simulink model "uvms_total"  (Simulink 8.1)
settings: Solver=ode23  StartTime=0.0  StopTime=2  FixedStep=dt  RelTol=1e-4
values from neighbouring files (symbols this model uses):
  DH = struct('a',zeros(n,1),'d',zeros(n,1),'alpha',zeros(n,1))    [init.m]
  dt = 0.01    [run_simulation.m]
undefined symbols (not defined in the file or in its folder): ee_pose_init, ee_pose_quaternion_init, KinematicControlParameters, Kinetics_Parameters, max_zeta, q_init, QLimits, reference_system_matrix_inv, reference_system_zeta_matrix_inv, V_current, vehicle_position_init, vehicle_quaternion_init, VV_States
(part 1 of 2)
settings Model: Creator=simena  LastModifiedBy=simena  SimulationMode=accelerator
settings SolverCC: ZeroCrossControl=DisableAll
settings DataIOCC: InspectSignalLogs=on
settings OptimizationCC: SimCompilerOptimization=On
settings DebuggingCC: AlgebraicLoopMsg=error  UnderspecifiedInitializationDetection=Simplified  FcnCallInpInsideContextMsg=EnableAllAsWarning
settings SFSimCC: SFSimEnableDebug=off
settings GRTTargetCC: CombineOutputUpdateFcns=on  GRTInterface=off

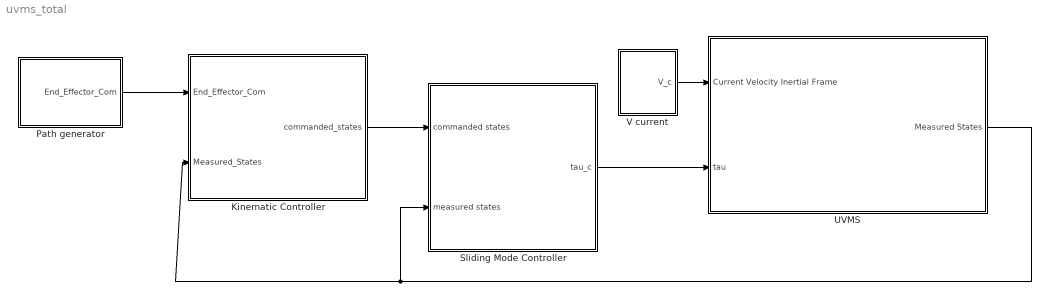
== system uvms_total ==
  Kinematic Controller : Subsystem
  Path generator : Subsystem
  Sliding Mode Controller : Subsystem
  UVMS : Subsystem
  V current : Subsystem
  wires:
  Sliding Mode Controller/1(tau_c) -> UVMS/2(tau)
  UVMS/1(Measured States) -> Sliding Mode Controller/2(measured states), Kinematic Controller/2(Measured_States)
  V current/1(V_c) -> UVMS/1(Current Velocity Inertial Frame)
  Path generator/1(End_Effector_Com) -> Kinematic Controller/1(End_Effector_Com)
  Kinematic Controller/1(commanded_states) -> Sliding Mode Controller/1(commanded states)

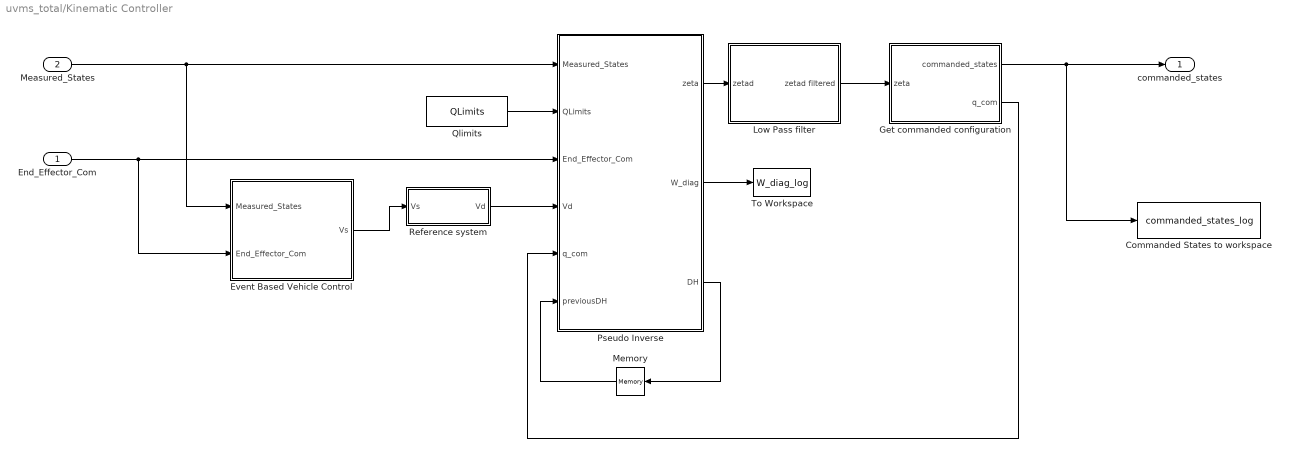
== system uvms_total/Kinematic Controller ==
  End_Effector_Com : Inport
  Measured_States : Inport  Port=2
  Commanded States to workspace : ToWorkspace  VariableName=commanded_states_log  SampleTime=dt  SaveFormat=Timeseries
  Event Based Vehicle Control : Subsystem
  Get commanded configuration : Subsystem  TreatAsAtomicUnit=on
  Low Pass filter : Subsystem
  Memory : Memory
  Pseudo Inverse : MATLAB Function  TreatAsAtomicUnit=on
  Qlimits : Constant  Value=QLimits  OutDataTypeStr=Bus: qlimits_bus
  Reference system : Subsystem
  To Workspace : ToWorkspace  VariableName=W_diag_log  SampleTime=dt  SaveFormat=Timeseries
  commanded_states : Outport
  wires:
  Qlimits/1 -> Pseudo Inverse/2(QLimits)
  Memory/1 -> Pseudo Inverse/6(previousDH)
  Event Based Vehicle Control/1(Vs) -> Reference system/1(Vs)
  Pseudo Inverse/2(W_diag) -> To Workspace/1
  Pseudo Inverse/3(DH) -> Memory/1
  Pseudo Inverse/1(zeta) -> Low Pass filter/1(zetad)
  Measured_States/1 -> Pseudo Inverse/1(Measured_States), Event Based Vehicle Control/1(Measured_States)
  Reference system/1(Vd) -> Pseudo Inverse/4(Vd)
  Get commanded configuration/2(q_com) -> Pseudo Inverse/5(q_com)
  Low Pass filter/1(zetad filtered) -> Get commanded configuration/1(zeta)
  Get commanded configuration/1(commanded_states) -> commanded_states/1, Commanded States to workspace/1
  End_Effector_Com/1 -> Pseudo Inverse/3(End_Effector_Com), Event Based Vehicle Control/2(End_Effector_Com)

== system uvms_total/Path generator ==
  EE velocity in frame 0 to EE velocity in frame e : MATLAB Function  TreatAsAtomicUnit=on
  End Effector2 : Subsystem
  From Workspace : FromWorkspace  VariableName=ee_traj_input  SampleTime=0
  To Workspace : ToWorkspace  VariableName=Ee_com_log  SampleTime=dt  SaveFormat=Timeseries
  End_Effector_Com : Outport
  wires:
  From Workspace/1 -> EE velocity in frame 0 to EE velocity in frame e/2(V0)  "v_ee_c_0"
  End Effector2/2(End Effector) -> End_Effector_Com/1, To Workspace/1
  EE velocity in frame 0 to EE velocity in frame e/1(Vb) -> End Effector2/1(v_ee_com)  "v_ee_c"
  End Effector2/1(ee_pose_euler) -> EE velocity in frame 0 to EE velocity in frame e/1(pose)

== system uvms_total/Sliding Mode Controller ==
  commanded states : Inport
  measured states : Inport  Port=2
  To Workspace1 : ToWorkspace  VariableName=tau_log  SampleTime=dt  SaveFormat=Timeseries
  sliding mode 2 : Subsystem
  tau_c : Outport
  wires:
  sliding mode 2/1(tau) -> To Workspace1/1, tau_c/1
  measured states/1 -> sliding mode 2/1(measured states)
  commanded states/1 -> sliding mode 2/2(commanded states)

== system uvms_total/UVMS ==
  Current Velocity Inertial Frame : Inport
  tau : Inport  Port=2
  Kinetics : Subsystem
      settings: MinAlgLoopOccurrences=on
  Log Measured States : Subsystem
  Measured States : Outport
  wires:
  tau/1 -> Kinetics/1(tau)
  Current Velocity Inertial Frame/1 -> Kinetics/2(Current Inertial Frame)
  Kinetics/1(measured_states) -> Log Measured States/1(measured_states), Measured States/1, Kinetics/3(Measured_States)

== system uvms_total/V current ==
  Current : Constant  Value=V_current
  V_c : Outport
  wires:
  Current/1 -> V_c/1

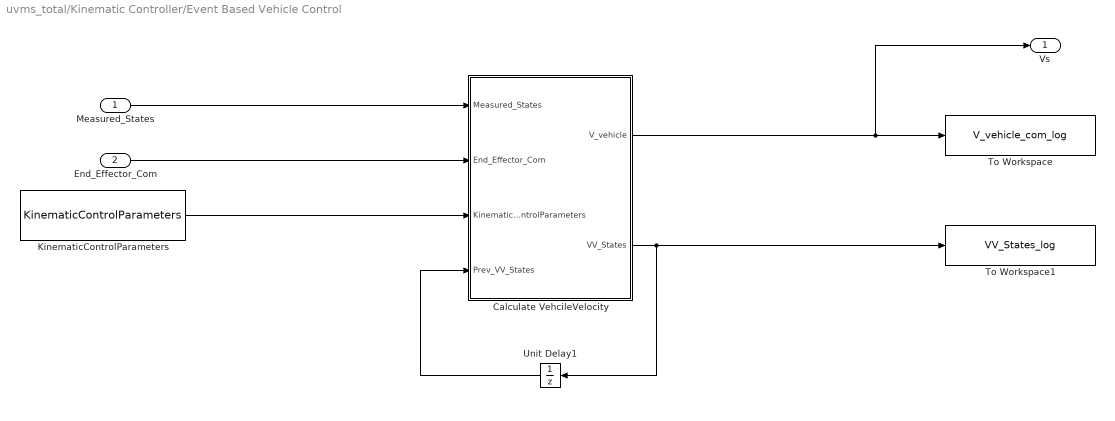
== system uvms_total/Kinematic Controller/Event Based Vehicle Control ==
  Measured_States : Inport
  End_Effector_Com : Inport  Port=2
  Calculate VehcileVelocity : MATLAB Function  TreatAsAtomicUnit=on  SystemSampleTime=dt
  KinematicControlParameters : Constant  Value=KinematicControlParameters  OutDataTypeStr=Bus: kinematicControlParameters_bus
  To Workspace : ToWorkspace  VariableName=V_vehicle_com_log  SampleTime=dt  SaveFormat=Timeseries
  To Workspace1 : ToWorkspace  VariableName=VV_States_log  SampleTime=dt  SaveFormat=Timeseries
  Unit Delay1 : UnitDelay  InitialCondition=VV_States  SampleTime=-1
  Vs : Outport
  wires:
  Unit Delay1/1 -> Calculate VehcileVelocity/4(Prev_VV_States)
  Measured_States/1 -> Calculate VehcileVelocity/1(Measured_States)
  End_Effector_Com/1 -> Calculate VehcileVelocity/2(End_Effector_Com)
  Calculate VehcileVelocity/2(VV_States) -> To Workspace1/1, Unit Delay1/1
  KinematicControlParameters/1 -> Calculate VehcileVelocity/3(KinematicControlParameters)
  Calculate VehcileVelocity/1(V_vehicle) -> Vs/1, To Workspace/1

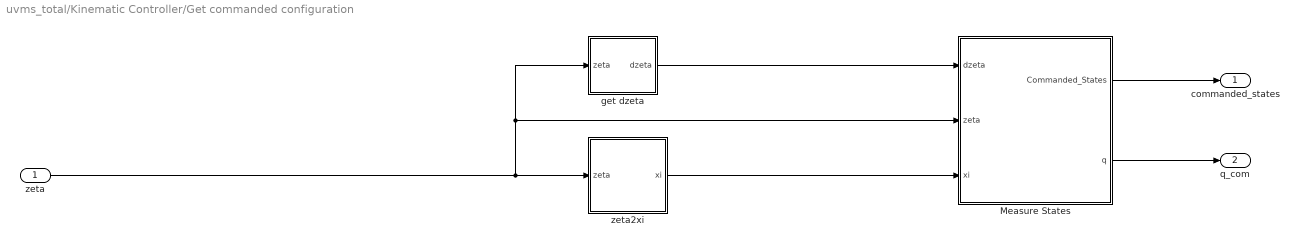
== system uvms_total/Kinematic Controller/Get commanded configuration ==
  zeta : Inport
  Measure States : MATLAB Function  TreatAsAtomicUnit=on
  get dzeta : Subsystem
  zeta2xi : Subsystem
  commanded_states : Outport
  q_com : Outport  Port=2
  wires:
  Measure States/1(Commanded_States) -> commanded_states/1
  zeta/1 -> zeta2xi/1(zeta), Measure States/2(zeta), get dzeta/1(zeta)
  get dzeta/1(dzeta) -> Measure States/1(dzeta)
  Measure States/2(q) -> q_com/1
  zeta2xi/1(xi) -> Measure States/3(xi)

== system uvms_total/Kinematic Controller/Low Pass filter ==
  zetad : Inport
  Integrator : Integrator
  Sum : Sum  Inputs=+-
  time constants : Gain  Gain=reference_system_zeta_matrix_inv  Multiplication=Matrix(K*u)
  zetad filtered : Outport
  wires:
  Sum/1 -> time constants/1
  Integrator/1 -> Sum/2, zetad filtered/1
  time constants/1 -> Integrator/1
  zetad/1 -> Sum/1

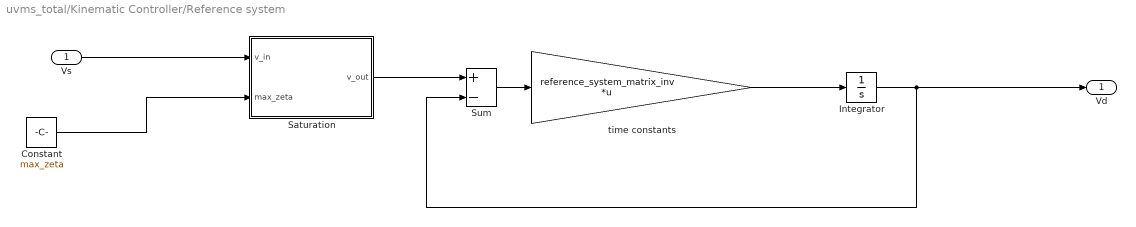
== system uvms_total/Kinematic Controller/Reference system ==
  Vs : Inport
  Constant : Constant  Value=max_zeta
  Integrator : Integrator  InitialCondition=zeros(6,1)
  Saturation : MATLAB Function  TreatAsAtomicUnit=on
  Sum : Sum  Inputs=+-
  time constants : Gain  Gain=reference_system_matrix_inv  Multiplication=Matrix(K*u)
  Vd : Outport
  wires:
  Sum/1 -> time constants/1
  Constant/1 -> Saturation/2(max_zeta)
  time constants/1 -> Integrator/1
  Saturation/1(v_out) -> Sum/1
  Vs/1 -> Saturation/1(v_in)
  Integrator/1 -> Vd/1, Sum/2

== system uvms_total/Path generator/End Effector2 ==
  v_ee_com : Inport
  MATLAB Function1 : MATLAB Function  TreatAsAtomicUnit=on
  twist2pose_euler : Subsystem
  twist2pose_quaternions : Subsystem
  ee_pose_euler : Outport
  End Effector : Outport  Port=2
  wires:
  MATLAB Function1/1(End_Effector_Com) -> End Effector/1
  v_ee_com/1 -> MATLAB Function1/1(velocity), twist2pose_euler/1(v_ee), twist2pose_quaternions/1(v_ee)
  twist2pose_euler/1(ee_pose) -> ee_pose_euler/1
  twist2pose_quaternions/1(ee_pose) -> MATLAB Function1/2(pose)

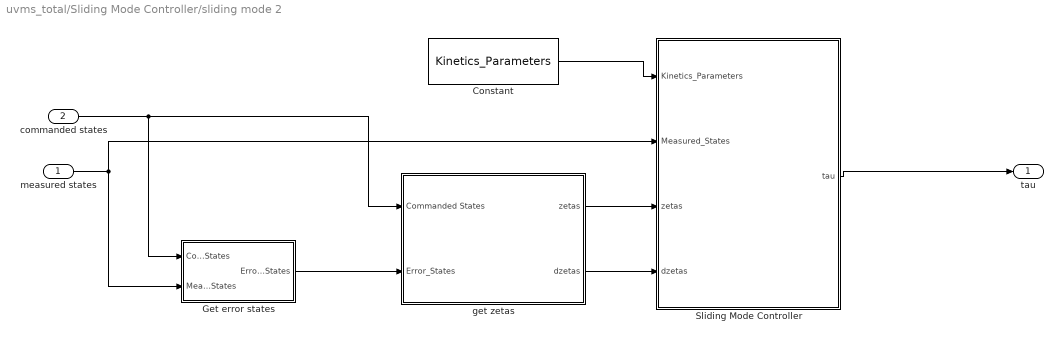
== system uvms_total/Sliding Mode Controller/sliding mode 2 ==
  measured states : Inport
  commanded states : Inport  Port=2
  Constant : Constant  Value=Kinetics_Parameters  OutDataTypeStr=Bus: kinetics_bus
  Get error states : Subsystem
  Sliding Mode Controller : MATLAB Function  TreatAsAtomicUnit=on
  get zetas : Subsystem
  tau : Outport
  wires:
  Constant/1 -> Sliding Mode Controller/1(Kinetics_Parameters)
  Sliding Mode Controller/1(tau) -> tau/1
  get zetas/1(zetas) -> Sliding Mode Controller/3(zetas)
  get zetas/2(dzetas) -> Sliding Mode Controller/4(dzetas)
  commanded states/1 -> get zetas/1(Commanded States), Get error states/1(Commanded States)
  measured states/1 -> Sliding Mode Controller/2(Measured_States), Get error states/2(Measured States)
  Get error states/1(Error States) -> get zetas/2(Error_States)

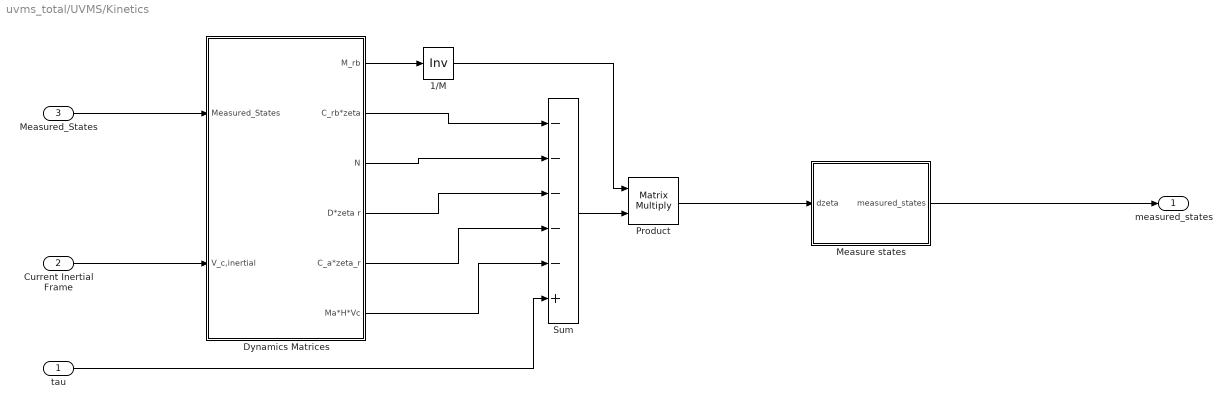
== system uvms_total/UVMS/Kinetics ==
  tau : Inport
  Current Inertial Frame : Inport  Port=2
  Measured_States : Inport  Port=3
  1/M : Product  Inputs=/  Multiplication=Matrix(*)
  Dynamics Matrices : Subsystem
  Measure states : Subsystem  TreatAsAtomicUnit=on
      settings: MinAlgLoopOccurrences=on
  Product : Product  Multiplication=Matrix(*)  RndMeth=Zero
  Sum : Sum  Inputs=-----+
  measured_states : Outport
  wires:
  Dynamics Matrices/1(M_rb) -> 1/M/1
  Sum/1 -> Product/2
  Product/1 -> Measure states/1(dzeta)
  Measure states/1(measured_states) -> measured_states/1
  1/M/1 -> Product/1
  Current Inertial Frame/1 -> Dynamics Matrices/2(V_c,inertial)
  Dynamics Matrices/2(C_rb*zeta) -> Sum/1
  Dynamics Matrices/3(N) -> Sum/2
  Dynamics Matrices/4(D*zeta r) -> Sum/3
  Dynamics Matrices/5(C_a*zeta_r) -> Sum/4
  Dynamics Matrices/6(Ma*H*Vc) -> Sum/5
  tau/1 -> Sum/6
  Measured_States/1 -> Dynamics Matrices/1(Measured_States)

== system uvms_total/UVMS/Log Measured States ==
  measured_states : Inport
  To Workspace1 : ToWorkspace  VariableName=measured_states_log  SampleTime=dt  SaveFormat=Timeseries
  wires:
  measured_states/1 -> To Workspace1/1

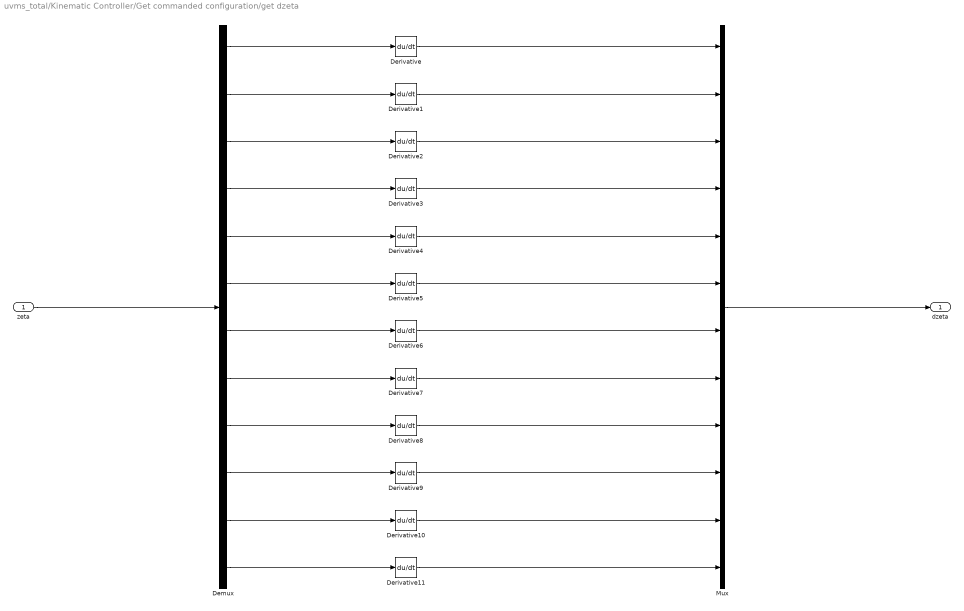
== system uvms_total/Kinematic Controller/Get commanded configuration/get dzeta ==
  zeta : Inport
  Demux : Demux  Outputs=12
  Derivative{,1..11} (12 alike) : Derivative
  Mux : Mux  Inputs=12
  dzeta : Outport
  wires:
  Demux/1 -> Derivative/1
  zeta/1 -> Demux/1
  Derivative/1 -> Mux/1
  Demux/2 -> Derivative1/1
  Demux/3 -> Derivative2/1
  Demux/4 -> Derivative3/1
  Demux/5 -> Derivative4/1
  Demux/6 -> Derivative5/1
  Demux/7 -> Derivative6/1
  Demux/8 -> Derivative7/1
  Demux/9 -> Derivative8/1
  Demux/10 -> Derivative9/1
  Demux/11 -> Derivative10/1
  Demux/12 -> Derivative11/1
  Derivative1/1 -> Mux/2
  Derivative2/1 -> Mux/3
  Derivative3/1 -> Mux/4
  Derivative4/1 -> Mux/5
  Derivative5/1 -> Mux/6
  Derivative6/1 -> Mux/7
  Derivative7/1 -> Mux/8
  Derivative8/1 -> Mux/9
  Derivative9/1 -> Mux/10
  Derivative10/1 -> Mux/11
  Derivative11/1 -> Mux/12
  Mux/1 -> dzeta/1

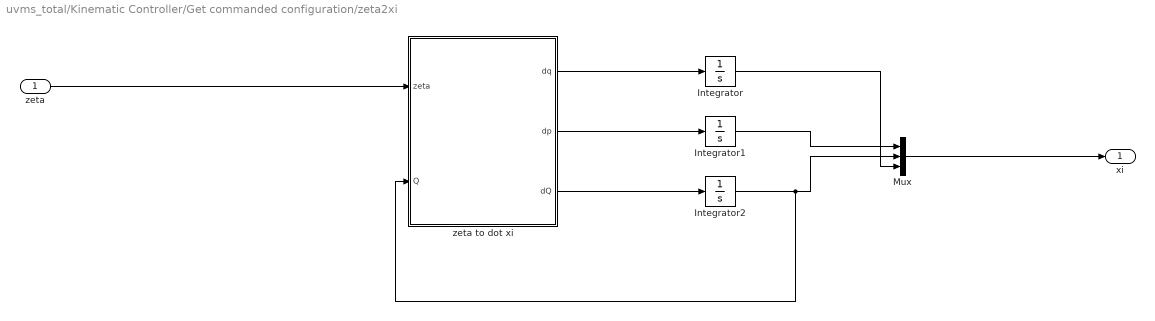
== system uvms_total/Kinematic Controller/Get commanded configuration/zeta2xi ==
  zeta : Inport
  Integrator : Integrator  InitialCondition=q_init
  Integrator1 : Integrator  InitialCondition=vehicle_position_init
  Integrator2 : Integrator  InitialCondition=vehicle_quaternion_init
  Mux : Mux  Inputs=3
  zeta to dot xi : MATLAB Function  TreatAsAtomicUnit=on
  xi : Outport
  wires:
  zeta to dot xi/1(dq) -> Integrator/1
  zeta to dot xi/2(dp) -> Integrator1/1
  zeta to dot xi/3(dQ) -> Integrator2/1
  zeta/1 -> zeta to dot xi/1(zeta)
  Mux/1 -> xi/1
  Integrator1/1 -> Mux/1
  Integrator2/1 -> Mux/2, zeta to dot xi/2(Q)
  Integrator/1 -> Mux/3

== system uvms_total/Path generator/End Effector2/twist2pose_euler ==
  v_ee : Inport
  Demux : Demux  Outputs=2
  Integrator : Integrator  InitialCondition=ee_pose_init
  Mux : Mux  Inputs=2
  body2eulervel : MATLAB Function  TreatAsAtomicUnit=on  SystemSampleTime=dt
  ee_pose : Outport
  wires:
  v_ee/1 -> body2eulervel/1(ee_velocity_twist)
  body2eulervel/1(ee_rates) -> Integrator/1
  Integrator/1 -> Demux/1
  Demux/2 -> body2eulervel/2(euler_angles_ee), Mux/2  "ee_angle"
  Demux/1 -> Mux/1  "ee_pos"
  Mux/1 -> ee_pose/1

== system uvms_total/Path generator/End Effector2/twist2pose_quaternions ==
  v_ee : Inport
  Integrator : Integrator  InitialCondition=ee_pose_quaternion_init
  MATLAB Function : MATLAB Function  TreatAsAtomicUnit=on
  body2quat : MATLAB Function  TreatAsAtomicUnit=on  SystemSampleTime=dt
  ee_pose : Outport
  wires:
  v_ee/1 -> body2quat/1(ee_velocity_twist)
  body2quat/1(ee_rates) -> Integrator/1
  Integrator/1 -> MATLAB Function/1(poseIn)
  MATLAB Function/1(pose) -> ee_pose/1
  MATLAB Function/2(quaternion) -> body2quat/2(quat)

== system uvms_total/Sliding Mode Controller/sliding mode 2/Get error states ==
  Commanded States : Inport
  Measured States : Inport  Port=2
  Log Error States : Subsystem
  MATLAB Function : MATLAB Function  TreatAsAtomicUnit=on
  Error States : Outport
  wires:
  Commanded States/1 -> MATLAB Function/1(Commanded_States)
  Measured States/1 -> MATLAB Function/2(Measured_States)
  MATLAB Function/1(Error_States) -> Log Error States/1(measured_states), Error States/1

== system uvms_total/Sliding Mode Controller/sliding mode 2/get zetas ==
  Commanded States : Inport
  Error_States : Inport  Port=2
  Derivative : Derivative  CoefficientInTFapproximation=0.01
  get dot y : MATLAB Function  TreatAsAtomicUnit=on
  zetas : Outport
  dzetas : Outport  Port=2
  wires:
  Commanded States/1 -> get dot y/1(Commanded_States)
  Error_States/1 -> get dot y/2(Error_States)
  get dot y/1(zetas) -> zetas/1, Derivative/1
  Derivative/1 -> dzetas/1

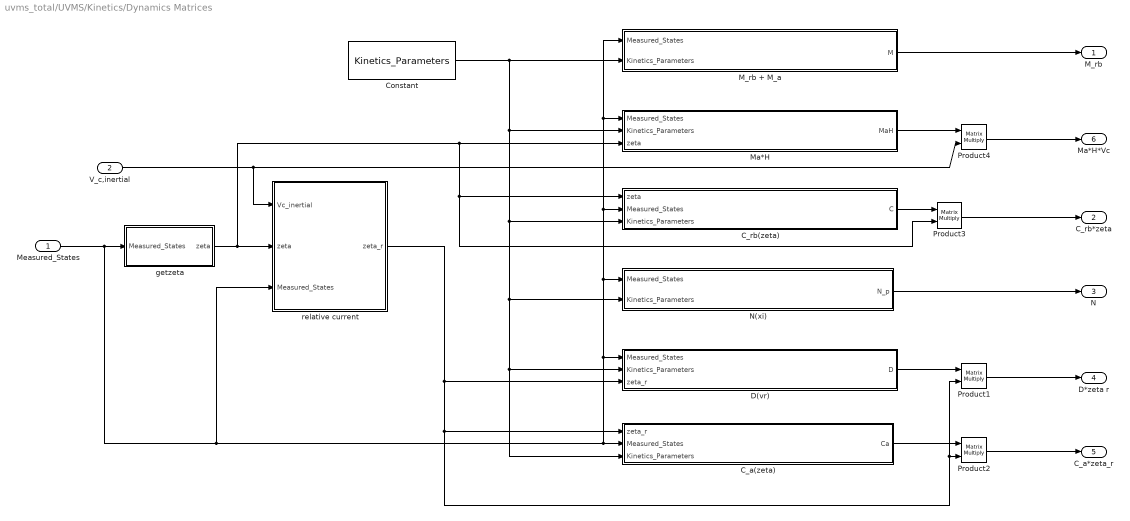
== system uvms_total/UVMS/Kinetics/Dynamics Matrices ==
  Measured_States : Inport
  V_c,inertial : Inport  Port=2
  C_a(zeta) : MATLAB Function  TreatAsAtomicUnit=on
  C_rb(zeta) : MATLAB Function  TreatAsAtomicUnit=on
  Constant : Constant  Value=Kinetics_Parameters  OutDataTypeStr=Bus: kinetics_bus
  D(vr) : MATLAB Function  TreatAsAtomicUnit=on
  M_rb + M_a : MATLAB Function  TreatAsAtomicUnit=on
  Ma*H : MATLAB Function  TreatAsAtomicUnit=on
  N(xi) : MATLAB Function  TreatAsAtomicUnit=on
  Product{1..4} (4 alike) : Product  Multiplication=Matrix(*)  RndMeth=Zero
  getzeta : MATLAB Function  TreatAsAtomicUnit=on
  relative current : MATLAB Function  TreatAsAtomicUnit=on
  M_rb : Outport
  C_rb*zeta : Outport  Port=2
  N : Outport  Port=3
  D*zeta r : Outport  Port=4
  C_a*zeta_r : Outport  Port=5
  Ma*H*Vc : Outport  Port=6
  wires:
  Product1/1 -> D*zeta r/1
  Product2/1 -> C_a*zeta_r/1
  Product3/1 -> C_rb*zeta/1
  M_rb + M_a/1(M) -> M_rb/1
  Ma*H/1(MaH) -> Product4/1
  relative current/1(zeta_r) -> D(vr)/3(zeta_r), C_a(zeta)/1(zeta_r), Product2/2, Product1/2
  Measured_States/1 -> relative current/3(Measured_States), C_a(zeta)/2(Measured_States), D(vr)/1(Measured_States), N(xi)/1(Measured_States), C_rb(zeta)/2(Measured_States), Ma*H/1(Measured_States), M_rb + M_a/1(Measured_States), getzeta/1(Measured_States)
  Constant/1 -> M_rb + M_a/2(Kinetics_Parameters), Ma*H/2(Kinetics_Parameters), C_rb(zeta)/3(Kinetics_Parameters), N(xi)/2(Kinetics_Parameters), C_a(zeta)/3(Kinetics_Parameters), D(vr)/2(Kinetics_Parameters)
  C_rb(zeta)/1(C) -> Product3/1
  N(xi)/1(N_p) -> N/1
  D(vr)/1(D) -> Product1/1
  C_a(zeta)/1(Ca) -> Product2/1
  V_c,inertial/1 -> Product4/2, relative current/1(Vc_inertial)
  Product4/1 -> Ma*H*Vc/1
  getzeta/1(zeta) -> relative current/2(zeta), Ma*H/3(zeta), C_rb(zeta)/1(zeta), Product3/2

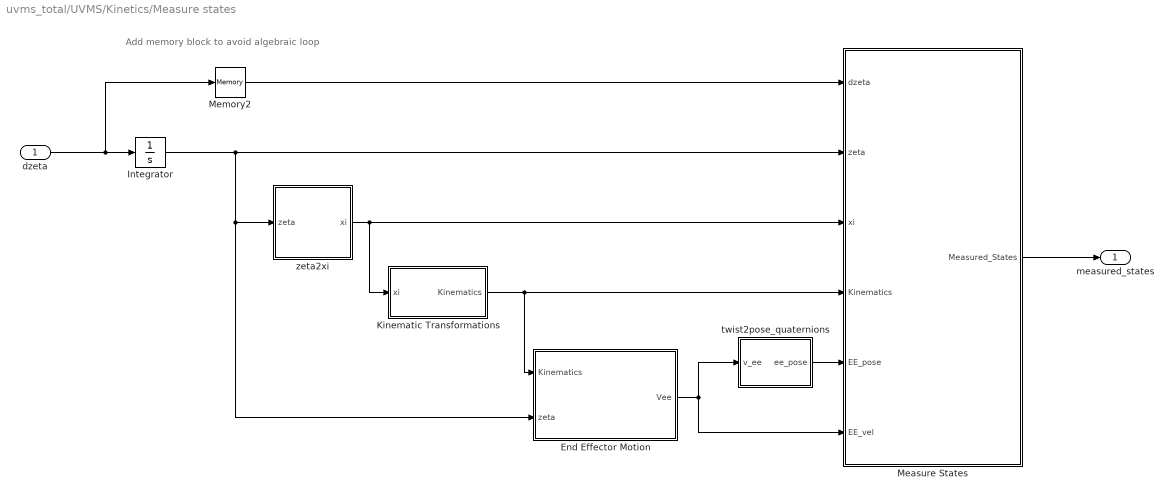
== system uvms_total/UVMS/Kinetics/Measure states ==
  note: Add memory block
      | to avoid algebraic
      | loop
  dzeta : Inport
  End Effector Motion : MATLAB Function  TreatAsAtomicUnit=on
  Integrator : Integrator
  Kinematic Transformations : Subsystem  SystemSampleTime=dt
      settings: MinAlgLoopOccurrences=on
  Measure States : MATLAB Function  TreatAsAtomicUnit=on
  Memory2 : Memory
  twist2pose_quaternions : Subsystem
  zeta2xi : Subsystem
  measured_states : Outport
  wires:
  Measure States/1(Measured_States) -> measured_states/1
  zeta2xi/1(xi) -> Measure States/3(xi), Kinematic Transformations/1(xi)
  Memory2/1 -> Measure States/1(dzeta)
  dzeta/1 -> Integrator/1, Memory2/1
  Integrator/1 -> End Effector Motion/2(zeta), zeta2xi/1(zeta), Measure States/2(zeta)
  twist2pose_quaternions/1(ee_pose) -> Measure States/5(EE_pose)
  End Effector Motion/1(Vee) -> Measure States/6(EE_vel), twist2pose_quaternions/1(v_ee)
  Kinematic Transformations/1(Kinematics) -> End Effector Motion/1(Kinematics), Measure States/4(Kinematics)

== system uvms_total/Sliding Mode Controller/sliding mode 2/Get error states/Log Error States ==
  measured_states : Inport
  To Workspace1 : ToWorkspace  VariableName=Error_States_log  SampleTime=dt  SaveFormat=Timeseries
  wires:
  measured_states/1 -> To Workspace1/1

== system uvms_total/UVMS/Kinetics/Measure states/Kinematic Transformations ==
  xi : Inport
  DH parameters : Constant  Value=DH  OutDataTypeStr=Bus: DH_bus
  Jacobians : MATLAB Function  TreatAsAtomicUnit=on
  Transformations : MATLAB Function  TreatAsAtomicUnit=on
  Kinematics : Outport
  wires:
  DH parameters/1 -> Transformations/2(DH)  "DH"
  Transformations/1(Ti) -> Jacobians/1(Ti)
  Jacobians/1(Kinematics) -> Kinematics/1
  xi/1 -> Transformations/1(xi)

== system uvms_total/UVMS/Kinetics/Measure states/twist2pose_quaternions ==
  v_ee : Inport
  Integrator : Integrator  InitialCondition=ee_pose_quaternion_init
  MATLAB Function : MATLAB Function  TreatAsAtomicUnit=on
  body2quat : MATLAB Function  TreatAsAtomicUnit=on
  ee_pose : Outport
  wires:
  v_ee/1 -> body2quat/1(ee_velocity_twist)
  body2quat/1(ee_rates) -> Integrator/1
  Integrator/1 -> MATLAB Function/1(poseIn)
  MATLAB Function/1(pose) -> ee_pose/1
  MATLAB Function/2(quaternion) -> body2quat/2(quat)

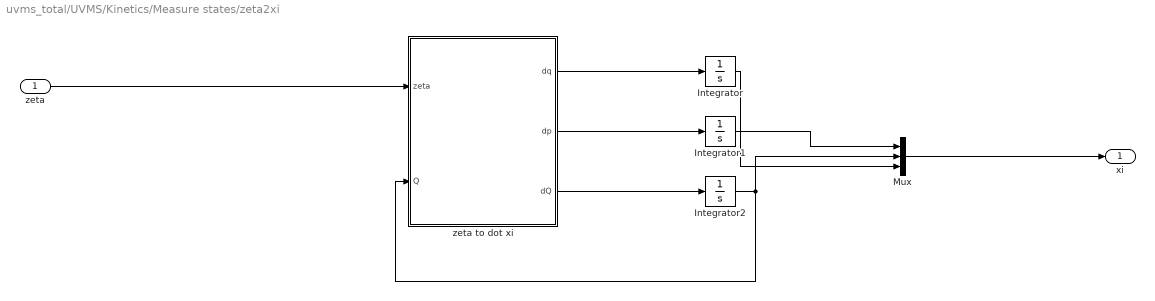
== system uvms_total/UVMS/Kinetics/Measure states/zeta2xi ==
  zeta : Inport
  Integrator : Integrator  InitialCondition=q_init
  Integrator1 : Integrator  InitialCondition=vehicle_position_init
  Integrator2 : Integrator  InitialCondition=vehicle_quaternion_init
  Mux : Mux  Inputs=3
  zeta to dot xi : MATLAB Function  TreatAsAtomicUnit=on  SystemSampleTime=dt
  xi : Outport
  wires:
  zeta to dot xi/1(dq) -> Integrator/1
  zeta to dot xi/2(dp) -> Integrator1/1
  zeta to dot xi/3(dQ) -> Integrator2/1
  zeta/1 -> zeta to dot xi/1(zeta)
  Integrator2/1 -> zeta to dot xi/2(Q), Mux/2
  Mux/1 -> xi/1
  Integrator1/1 -> Mux/1
  Integrator/1 -> Mux/3

== matlab function UVMS/Kinetics/Measure states/Kinematic Transformations/Jacobians ==
  data: Ti input Bus: Ti_bus; Kinematics output Bus: kin_bus
function Kinematics  = getJacobians(Ti)
%#codegen
    n=6;
    Ji = struct('Ji',zeros(n,n+6,n),'Je',zeros(n,n+6),'Jbe',zeros(n,n));
    Kinematics = struct('Ti', Ti, 'Ji',Ji);
    ji=zeros(6,6);
    for i=1:n
        ji=getji(Ti,i);
    
        Ji.Ji(:,:,i) = [Ti.Adgbi_inv(:,:,i), Ti.Adgbi_inv(:,:,i)*ji];
    end
    j6 = getje(Ti);
    Ji.Je = [Ti.Adgbe_inv, Ti.Adgbe_inv*j6];
    Ji.Jbe = Ti.Adgbe_inv*j6;
    Kinematics.Ji = Ji;
    Kinematics.Ti = Ti;
end




% return matrix Ji (see report)
function mat = getji(Ti,i)
    n=6;
    mat=zeros(6,6);
    Xii=[0,0,0,0,0,1]';
    mat(:,1)=eye(6)*Xii;
    for j=2:n
        if j<=i
            mat(:,j) = Ti.Adgbi(:,:,j-1)*Xii;
        end
    end

end

% return matrix Je (see report)
function mat = getje(Ti)
    n=6;
    mat=zeros(6,6);
    Xii=[0,0,0,0,0,1]';
    mat(:,1)=eye(6)*Xii;
    for i=2:(n-1)
        mat(:,i) = Ti.Adgbi(:,:,i-1)*Xii;
    end
    mat(:,6) = Ti.Adgbe*Xii;

end

== matlab function UVMS/Kinetics/Measure states/Kinematic Transformations/Transformations ==
  data: xi input double; DH input Bus: DH_bus; Ti output Bus: Ti_bus
function Ti = getTransformations(xi,DH)
%#codegen
% Return transformations, rotations, positions and adjoint matrices for
% robot links
% Tbi.gbi(:,:,i) is the transformation from b to i etc
    n = 6;    % number of links
    %xi = Measured_States.xi;
    q = xi(8:13);
    eta = xi(1:7);
    Q = eta(4:7);
    x = eta(1:3);
    Ti = struct('g0b',zeros(4,4),'g0i',zeros(4,4,n),'R0i', zeros(3,3,n),'R0b',zeros(3,3),'p0i', zeros(3,1,n),  'Adg0i',zeros(6,6,n),'Adg0i_inv',zeros(6,6,n),   ...
    'gbi',zeros(4,4,n),'Rbi', zeros(3,3,n),'pbi', zeros(3,1,n),'Adgbi',zeros(6,6,n),'Adgbi_inv',zeros(6,6,n),...
    'g6e', eye(4) ,'g0e',zeros(4,4),'R0e', zeros(3,3),'p0e', zeros(3,1),  'Adg0e',zeros(6,6),'Adg0e_inv',zeros(6,6),   ...
    'gbe',zeros(4,4),'Rbe', zeros(3,3),'pbe', zeros(3,1),'Adgbe',zeros(6,6),'Adgbe_inv',zeros(6,6) ...
    );
        
    Ti.g0b = eta2g0b(eta);
    Ti.R0b = Ti.g0b(1:3,1:3);

    % initial matrices 
    g = eye(4);
    g0 = Ti.g0b;
    
    for xi = 1:n
       % transformations from frame b to frame i
       Ti.gbi(:,:,xi) = g*getHom(q,DH,xi);
       Ti.Rbi(:,:,xi) = getRot(Ti.gbi(:,:,xi));
       Ti.pbi(:,:,xi) = getPos(Ti.gbi(:,:,xi));
       Ti.Adgbi(:,:,xi) = getAdgbi(Ti.Rbi(:,:,xi), Ti.pbi(:,:,xi) );
       Ti.Adgbi_inv(:,:,xi) = getAdgbi_inv(Ti.Rbi(:,:,xi), Ti.pbi(:,:,xi) );
       g = Ti.gbi(:,:,xi);
       % transformations from frame 0 to frame i
       Ti.g0i(:,:,xi) = g0*getHom(q,DH,xi);
       Ti.R0i(:,:,xi) = getRot(Ti.g0i(:,:,xi));
       Ti.p0i(:,:,xi) = getPos(Ti.g0i(:,:,xi));
       Ti.Adg0i(:,:,xi) = getAdgbi(Ti.R0i(:,:,xi), Ti.p0i(:,:,xi) );
       Ti.Adg0i_inv(:,:,xi) = getAdgbi_inv(Ti.R0i(:,:,xi), Ti.p0i(:,:,xi) );
       g0 = Ti.g0i(:,:,xi);
    end
    
    % transformation from frame 0 to ee
    g0e = Ti.g0i(:,:,6)*Ti.g6e;
    Ti.g0e = g0e;
    Ti.R0e = getRot(g0e);
    Ti.p0e = getPos(g0e);
    Ti.Adg0e = getAdgbi(Ti.R0e, Ti.p0e );
    Ti.Adg0e_inv = getAdgbi_inv(Ti.R0e, Ti.p0e);
        
    % transformation from frame b to ee
    gbe = Ti.gbi(:,:,6)*Ti.g6e;
    Ti.gbe = gbe;
    Ti.Rbe = getRot(gbe);
    Ti.pbe = getPos(gbe);
    Ti.Adgbe = getAdgbi(Ti.Rbe , Ti.pbe );
    Ti.Adgbe_inv = getAdgbi_inv(Ti.Rbe , Ti.pbe );
        
 end

% homogenous transformation matrix - DH convention
% mat = Rot_z(theta)Trans_z(d)Trans_x(a)Rot_x(alpha)
function mat = getHom(q,DH,i)
    alpha = DH.alpha(i);
    a = DH.a(i);
    d = DH.d(i);
    theta = q(i);
    mat = eye(4);
    mat = [cos(theta), -sin(theta)*cos(alpha), sin(theta)*sin(alpha), a*cos(theta);
         sin(theta), cos(theta)*cos(alpha), -cos(theta)*sin(alpha), a*sin(theta);
         0, sin(alpha), cos(alpha), d;
         0,0,0,1
    ];
end

% extract position from homogenous 
% matrix
function vec = getPos(g)
    vec = g(1:3,4);
end

% extract rotation matrix-part out of
% homogenous matrix
function mat = getRot(g)
    mat = g(1:3,1:3);
end

function mat = getAdgbi(R,p)
    ps = skew(p);
    mat = [R , ps*R ; zeros(3,3), R ];
end

function mat = getAdgbi_inv(R,p)
    Rt = transpose(R);
    ps = skew(p);
    mat = [Rt , -Rt*ps ; zeros(3,3), Rt ];
end

function mat = eta2g0b(eta)
    R = Rquat(eta(4:7));
    pos = [eta(1); eta(2); eta(3)];
    mat = [R,pos;0,0,0,1];
end

%-----------------------------------------------
% get rotation matrix from quaternion
function R = Rquat(Q)
    tol = 5*1e-2;
    if abs(norm(Q)-1)>tol 
        Q
        norm(Q)
        error('norm(q) must be equal to 1 (in get transformations) Try decreasing sampling time');
    end
    eta = Q(1);
    eps = Q(2:4);
    S = skew(eps);
    R = eye(3) + 2*eta*S + 2*S^2;
end

== matlab function Kinematic Controller/Pseudo Inverse ==
  data: Measured_States input Bus: measured_states_bus; QLimits input Bus: qlimits_bus; zeta output double size=12; W_diag output double; End_Effector_Com input double; Vd input double; q_com input double; previousDH input double; DH output double size=12,12
function [zeta, W_diag, DH] = getZeta(Measured_States, QLimits, End_Effector_Com, Vd , q_com , previousDH)
%
%  Vp is the primary task trajectory - end effector
%  Vs is the secondary task trajectory - vehicle
%
%#codegen
    Jp = Measured_States.Ji.Je;
    Js = [eye(6), zeros(6,6)];
    q = q_com;
    Vp = End_Effector_Com.velocity;
    [W, DH] = getW(q,previousDH,QLimits);
    JpInv = zeros(12,6);
    JsInv = zeros(12,6);
    JsInv(:,:) = Js' ; 
    JpInv(:,:) = W \ transpose(Jp) /((Jp /W) *transpose(Jp));
    I = eye(12);
    zeta = JpInv*(Vp  ) + ( I - JpInv*Jp) * JsInv * Vd;
    W_diag = diag(W);
end

% --------------------------------------------------------------------------
%   Returns the weighting matrix for use in the weighted pseudo inverse
% --------------------------------------------------------------------------
function [W, DH] = getW(q, previousDH,QLimits)
%#codegen    
% link joints
    DH =diag([zeros(1,6),zeros(1,6)]); % derivative of H matrix
    qmin = QLimits.qmin;
    qmax = QLimits.qmax;
    for i=1:6
        temp = (((qmax(i)-qmin(i)).^2)*(2*q(i)-qmax(i)-qmin(i))) ./ ((4*(qmax(i)-q(i)).^2) * ((q(i)-qmin(i)).^2));
        if (abs(temp) - abs(previousDH(i+6,i+6))) < 0 
            DH(i+6,i+6) = 0.97 * previousDH(i+6, i+6);
         else
            DH(i+6,i+6) = temp;
        end
   end
   % vehicle weights
   Kv = 4000;
   for i=1:6
      DH(i,i) =  Kv ;
   end
   W = eye(12);
   W = W + abs(DH);
   
end

== matlab function UVMS/Kinetics/Dynamics Matrices/M_rb + M_a ==
  data: Measured_States input Bus: measured_states_bus; M output double size=12,12; Kinetics_Parameters input Bus: kinetics_bus
function M = getInertiaMatrix(Measured_States, Kinetics_Parameters)
%#codegen
%   getInertiaMatrix Returns the sum of the Rigid body inertia and the added mass:
%   M_rb + M_a
%   
    n=6;
    i=1;
    M = zeros(12,12);
    Inertia = Kinetics_Parameters.Inertia;
    AddedInertia = Kinetics_Parameters.AddedInertia;
    Jgb = [eye(6), zeros(6,6)];                                 % Jacobian from vehicle 
    Ji=Jgb;
    Hi = Kinetics_Parameters.Persistent.Adgici(:,:,i);
    Ii=Hi'*(Inertia(:,:,1) + AddedInertia(:,:,1))*Hi;           % Inertia of vehicle in CO
    M=M+(Ji')*Ii*Ji;
    for i=1:n
        Ji = Measured_States.Ji.Ji(:,:,i);                           % body jacobian
        Hi =Kinetics_Parameters.Persistent.Adgici(:,:,i+1);        % get Transformation matrix of link i
        Ii=Hi'*(Inertia(:,:,i+1) + AddedInertia(:,:,i+1))*Hi;   % Transform Inertia matrix from CG to CO
        M=M+(Ji')*Ii*Ji;                                        % Add link i's inertia to total inertia
    end   
end

== matlab function UVMS/Kinetics/Dynamics Matrices/C_rb(zeta) ==
  data: zeta input double size=12; C output double; Measured_States input Bus: measured_states_bus; Kinetics_Parameters input Bus: kinetics_bus
function C = Coriolis(zeta,Measured_States,Kinetics_Parameters)
%-----------------------------------------------------------------------
%#codegen
%
%   This function calculates the coriolis according to From and Pettersen
%   (2013).
%-----------------------------------------------------------------------
    n=6;
    C=zeros(12,12);
    Inertia=Kinetics_Parameters.Inertia;
    Jis = Measured_States.Ji.Ji;
    
    % i = b
    Jgb = [eye(6), zeros(6,6)];
    i=1;
    Hi = Kinetics_Parameters.Persistent.Adgici(:,:,i);
    Ii=Hi'*Inertia(:,:,i);
    Wb = getWb(Ii,zeta);
    C = - (Jgb')*Wb*Hi*Jgb;     % time derivative of Jgb = 0  
    
    % i >=1
    for i=1:n
        Hi = Kinetics_Parameters.Persistent.Adgici(:,:,i+1);
        Ii=Hi'*Inertia(:,:,i+1);
        Wi=getWi(Ii,Jis(:,:,i), zeta);
        Jgi_dot=getJgi_dot(Measured_States, zeta,i);
        Jgi = Jis(:,:,i);
        
        C = C + (Jgi')*Ii*Hi*Jgi_dot - (Jgi')*Wi*Hi*Jgi;
    end
end



function Wb = getWb(I , zeta)
% Get the matrix Wi for i=b
% I: Inertia matrix for vehicle
% zeta: generalized velocity
    Wb = zeros(6,6);
    v = zeta(1:3);
    omega = zeta(4:6);
    mI = I(1:3,1:3); % Identity matrix times mass of link b
    Ib = I(4:6,4:6); % Moment of inertia
    mrgb = I(4:6,1:3); % mass times skew symmetric r_g^b
    dKv= mI*v - mrgb*omega;
    dKomega = Ib*omega + mrgb*v;
    
    Wb = [zeros(3,3), skew(dKv) ; skew(dKv), skew(dKomega)];
end

function Wi = getWi(I, Ji,zeta)
% Get matrix Wi for robot links
% I: inertia matrix for link i
% Ji: Jacobian for link i
% zeta: generalized coordinates
    Wi = zeros(6,6);
    V0i = Ji*zeta;
    v = V0i(1:3);
    omega = V0i(4:6);
    mI = I(1:3,1:3); % Identity matrix times mass of link b
    Ib = I(4:6,4:6); % Moment of inertia
    mrgb = I(4:6,1:3); % mass times skew symmetric r_g^b
    dKv= mI*v - mrgb*omega;
    dKomega = Ib*omega + mrgb*v;
    Wi = [zeros(3,3), skew(dKv) ; skew(dKv), skew(dKomega)];
end

function Jgi_dot=getJgi_dot(Kinematics, zeta,i)
% the functions below is related to Jgi_dot
    Jgi_dot = zeros(6,6+6);
    n=6;
    Jgi = Kinematics.Ji.Ji(:,:,i);
    omega = Jgi*zeta;
    Rbi = Kinematics.Ti.Rbi(:,:,i);
    pbi = Kinematics.Ti.pbi(:,i);
    omegaib = getOmegaib(Kinematics,zeta,i);
    dpbi =  getDpbi(Kinematics,zeta,i);
        
    dAdg_inv = [(Rbi')*skew(omegaib) , -(Rbi')*skew(omegaib)*skew(pbi) + (Rbi')*skew(dpbi); ...
                zeros(3,3) , (Rbi')*skew(omegaib) ];
    dJi = zeros(6,6);
    omega0b = zeta(4:6);
    
    % get d/dt(Ji)
    Xii=[0,0,0,0,0,1]';
    for k=2:n
       if k<=i
            dpbk = getDpbi(Kinematics, zeta ,k-1);
            Rbk= Kinematics.Ti.Rbi(:,:,k-1);
            omega0k = [zeros(3,3) , eye(3)]*Kinematics.Ji.Ji(:,:,k-1)*zeta;
            omegabk = omega0k - (Rbk')*omega0b;
            dJi(:,k) = [zeros(3,3), skew(dpbk)*Rbk*skew(omegabk) ...
                ; zeros(3,3) , (Rbk')*skew(omegabk)]*Xii;
       end
    end
    Ji=getji(Kinematics.Ti, i);
    Adg_inv = Kinematics.Ti.Adgbi_inv(:,:,i);
    Jgi_dot = [dAdg_inv, dAdg_inv*Ji + Adg_inv*dJi ];
end

function omegaib = getOmegaib(Kinematics,zeta,i)
% returns angular rage of vehcile wrt frame i noted in vehicle frame
    omegaib = zeros(3,1);
    Rbi = Kinematics.Ti.Rbi(:,:,i);
    Jgi = Kinematics.Ji.Ji(:,:,i);
    omega0b = zeta(4:6);
    omegaib = omega0b - Rbi*[zeros(3,3), eye(3)]*Jgi*zeta;
end

function dpbi = getDpbi( Kinematics, zeta,iter)
% returns time derivative of position vector of from frame b to frame i
    dpbi = zeros(3,1);
    H = [eye(3), zeros(3,3)];
    Rbi=Kinematics.Ti.Rbi(:,:,iter);
    Adgbi_inv = Kinematics.Ti.Adgbi_inv(:,:,iter);
    Ji = getji(Kinematics.Ti,iter);
    qd=zeros(6,1);
    qd(:,:)=zeta(7:12);
    dpbi = Rbi*H*Adgbi_inv*Ji*qd;
end


function mat = getji(Ti,i)
% return matrix Ji (see report)
    n=6;
    mat=zeros(6,6);
    Xii=[0,0,0,0,0,1]';
    mat(:,1)=eye(6)*Xii;
    for j=2:n
        if j<=i
            mat(:,j) = Ti.Adgbi(:,:,j-1)*Xii;
        end
    end
end

function S = skew(v)
  S = [  0   -v(3)  v(2)
       v(3)  0    -v(1)
       -v(2) v(1)   0];
end

== matlab function UVMS/Kinetics/Dynamics Matrices/N(xi) ==
  data: Measured_States input Bus: measured_states_bus; N_p output double; Kinetics_Parameters input Bus: kinetics_bus
function N_p = Persistent_Forces(Measured_States,Kinetics_Parameters)
%#codegen
%   N_p - 12 x 1 vector of generalized forces
%   Persistent_Forces returns the generalized forces due to boyancy and 
%   gravity

    %% init
    n=6;
    N_p=zeros(12,1);
    Jgis = Measured_States.Ji.Ji;
    
    %%  vehicle
    F_bp = getFbp(Measured_States, Kinetics_Parameters,1);           % Get wrench from persistent forces in CO
    Jbb=([eye(6), zeros(6,6)]);                                 % Jacobian from b to b
    N_p = Jbb'*F_bp;                                            % Get contribution to total forces through Jbb
    
    %% robot links
    for i=1:n
        Jgi=Jgis(:,:,i);                                        % Jacobian from b to i
        F_ip = getFip(Measured_States,Kinetics_Parameters, i+1);     % Get wrench in CO
        N_p = N_p + (Jgi')*F_ip;                                % Map to generalized forces and add to total
    end
    N_p = - N_p;                                                % reverse the sign to comply with the sign convention
end
    
    
function F_ip = getFip(Kinematics,Kinetics_Parameters, i)
% function calculating wrench from persistent forces 
% i=b: vehicle
% i>=1: robot arms
    F_ip = zeros(6,1);
    mi = Kinetics_Parameters.Persistent.m(i);
    g = Kinetics_Parameters.Persistent.g;
    rho = Kinetics_Parameters.Persistent.rho;
    nabla = Kinetics_Parameters.Persistent.nabla(i);
    Ri0 = Kinematics.Ti.R0i(:,:,i-1)';
    Adgici = Kinetics_Parameters.Persistent.Adgici(:,:,i);  
    Adgibi = Kinetics_Parameters.Persistent.Adgibi(:,:,i);
    ez=[0;0;1];
    F_ip(:,:) = (Adgici')*[-mi*g*Ri0*ez ;0;0;0]  + (Adgibi')*[rho*nabla*g*Ri0*ez ;0;0;0 ];
end


function F_bp = getFbp(Kinematics,Kinetics_Parameters, i)
% function calculating wrench from persistent forces 
% i=b: vehicle
% i>=1: robot arms
    F_bp = zeros(6,1);
    mi = Kinetics_Parameters.Persistent.m(i);
    g = Kinetics_Parameters.Persistent.g;
    Adgici = Kinetics_Parameters.Persistent.Adgici(:,:,i);  
    Adgibi = Kinetics_Parameters.Persistent.Adgibi(:,:,i);
    rho = Kinetics_Parameters.Persistent.rho;
    nabla = Kinetics_Parameters.Persistent.nabla(i);
    Ri0 = (Kinematics.Ti.R0b)';
    ez=[0;0;1];
    F_bp(:,:) = (Adgici')*[-mi*g*Ri0*ez ; 0;0;0]  + (Adgibi')*[rho*nabla*g*Ri0*ez ; 0;0;0 ];
end



function [phi,theta,psi] = myR2euler(R)
    phi   = atan2(R(3,2),R(3,3));
    theta = -asin(R(3,1));
    psi   = atan2(R(2,1),R(1,1));
end

== matlab function UVMS/Kinetics/Dynamics Matrices/relative current ==
  data: Vc_inertial input double; zeta input double; Measured_States input Bus: measured_states_bus; zeta_r output double
function zeta_r  = getRealtiveCurrent(Vc_inertial,zeta,Measured_States)
%#codegen

    %% init
    R0b = Measured_States.Ti.R0b;
    omega_0b = zeta(4:6);
    vc = Vc_inertial(1:3);


    %% get zeta relative of the current
    VcB =  [R0b'*vc;zeros(3,1)];
    zeta_r = zeta - [VcB; zeros(6,1)];
end

== matlab function UVMS/Kinetics/Dynamics Matrices/D(vr) ==
  data: Measured_States input Bus: measured_states_bus; D output double; Kinetics_Parameters input double; zeta_r input double
function D = fcn(Measured_States, Kinetics_Parameters,zeta_r)
%#codegen
%
% Returns the D matrix in the dynamics equation. The total forces is based
% on mappin the forces in each frame to the total generalized forces
% through the jacoian: tau = J^T*F_i. The forces in frame i is calculated
% from the forces in CG to CO through the transformation matrix: F_co =
% Adgici^T*F_cg
%
    %% init
    n=6;
    D=zeros(12,12);                                      % init matrix size
    HydroDynamics = Kinetics_Parameters.HydroDynamics;   % Hydrodynamics parameters
    Jgis = Measured_States.Ji.Ji;                             % Jacobians
    Adgicis = Kinetics_Parameters.Persistent.Adgici;           % Transformation matrix
    
    
    %% vehicle
    i=1;
    Jbb=[eye(6), zeros(6)];                               % Jacobian from frame 0 to frame b
    Adgici = Adgicis(:,:,i);                                    % Transformation matrix
    Vcg = Adgici*Jbb*zeta_r;                                   % velocity in CG mapped from CO
    Dcg =  HydroDynamics.Linear(:,:,i) + ...
           HydroDynamics.Quadratic(:,:,i)*diag(abs(Vcg)); % Wrench in CG
    Di = Adgici'*Dcg;                                        % Wrench in CO mapped from CG    
    D = Jbb'*Di*Jbb;                                      % Add contribution to the total matrix mapped from frame i 
                                                          % to generalized coordinates                                   
    
    %% robot links
    for i=1:n
        Jgi = Jgis(:,:,i);                                % Jacobian from frame 0 to frame i 
        Adgici = Adgicis(:,:,i+1);                              % Transformation matrix
        Vcg = Adgici*Jgi*zeta_r;                               % velocity in CG
        Dcg = HydroDynamics.Linear(:,:,i+1)+... 
          HydroDynamics.Quadratic(:,:,i+1)*diag(abs(Vcg));% Wrench in CG   
        Di = Adgici'*Dcg;                                    % Wrench in CO    
        D = D + Jgi'*Di*Jgi;                              % Add frame i's contribution to D matrix    
    end

end

== matlab function UVMS/Kinetics/Measure states/Measure States ==
  data: dzeta input double; Measured_States output Bus: measured_states_bus; zeta input double; xi input double; Kinematics input double; EE_pose input double; EE_vel input double
function Measured_States = fcn(dzeta, zeta, xi, Kinematics, EE_pose, EE_vel)
%#codegen

Measured_States.dzeta = dzeta;
Measured_States.zeta = zeta;
Measured_States.xi = xi;
Measured_States.xi_euler = zeros(12,1);
Measured_States.Ti = Kinematics.Ti;
Measured_States.Ji = Kinematics.Ji;
Measured_States.EE_pose = EE_pose;
Measured_States.EE_velocity = EE_vel;

end

== matlab function UVMS/Kinetics/Dynamics Matrices/C_a(zeta) ==
  data: zeta_r input double size=12; Ca output double; Measured_States input Bus: measured_states_bus; Kinetics_Parameters input Bus: kinetics_bus
function Ca = AddedCoriolis(zeta_r,Measured_States,Kinetics_Parameters)
%#codegen ..............................................
%
%   This function calculates the added coriolis matrix
%.......................................................
    n=6;
    Ca=zeros(12,12);
    Inertia=Kinetics_Parameters.AddedInertia;
    Jis = Measured_States.Ji.Ji;
    
    % vehicle
    Jgb = [eye(6), zeros(6,6)];
    i=1;
    Hi = Kinetics_Parameters.Persistent.Adgici(:,:,i+1);
    Ii=Hi'*Inertia(:,:,i);
    Wb = getWb(Ii,zeta_r);
    Ca = - (Jgb')*Wb*Hi*Jgb;     % time derivative of Jgb = 0  
    
    % manipulator links
    for i=1:n
        Hi = Kinetics_Parameters.Persistent.Adgici(:,:,i+1);
        Ii=Hi'*Inertia(:,:,i+1);
        Wi=getWi(Ii,Jis(:,:,i), zeta_r);
        Jgi_dot=getJgi_dot(Measured_States, zeta_r,i);
        Jgi = Jis(:,:,i);
        Ca = Ca + (Jgi')*Ii*Hi*Jgi_dot - (Jgi')*Wi*Hi*Jgi;
    end
end



function Wb = getWb(I , zeta)
% Get the matrix Wi for i=b
% I: Inertia matrix for vehicle
% zeta: generalized velocity
    Wb = zeros(6,6);
    v = zeta(1:3);
    omega = zeta(4:6);
    mI = I(1:3,1:3); % Identity matrix times mass of link b
    Ib = I(4:6,4:6); % Moment of inertia
    mrgb = I(4:6,1:3); % mass times skew symmetric r_g^b
    dKv= mI*v - mrgb*omega;
    dKomega = Ib*omega + mrgb*v;
    
    Wb = [zeros(3,3), skew(dKv) ; skew(dKv), skew(dKomega)];
end

function Wi = getWi(I, Ji,zeta)
% Get matrix Wi for robot links
% I: inertia matrix for link i
% Ji: Jacobian for link i
% zeta: generalized coordinates
    Wi = zeros(6,6);
    V0i = Ji*zeta;
    v = V0i(1:3);
    omega = V0i(4:6);
    mI = I(1:3,1:3); % Identity matrix times mass of link b
    Ib = I(4:6,4:6); % Moment of inertia
    mrgb = I(4:6,1:3); % mass times skew symmetric r_g^b
    dKv= mI*v - mrgb*omega;
    dKomega = Ib*omega + mrgb*v;
    Wi = [zeros(3,3), skew(dKv) ; skew(dKv), skew(dKomega)];
end

function Jgi_dot=getJgi_dot(Kinematics, zeta,i)
% the functions below is related to Jgi_dot
    Jgi_dot = zeros(6,6+6);
    n=6;
    Jgi = Kinematics.Ji.Ji(:,:,i);
    omega = Jgi*zeta;
    Rbi = Kinematics.Ti.Rbi(:,:,i);
    pbi = Kinematics.Ti.pbi(:,i);
    omegaib = getOmegaib(Kinematics,zeta,i);
    dpbi =  getDpbi(Kinematics,zeta,i);
        
    dAdg_inv = [(Rbi')*skew(omegaib) , -(Rbi')*skew(omegaib)*skew(pbi) + (Rbi')*skew(dpbi); ...
                zeros(3,3) , (Rbi')*skew(omegaib) ];
    dJi = zeros(6,6);
    omega0b = zeta(4:6);
    
    % get d/dt(Ji)
    Xii=[0,0,0,0,0,1]';
    for k=2:n
       if k<=i
            dpbk = getDpbi(Kinematics, zeta ,k-1);
            Rbk= Kinematics.Ti.Rbi(:,:,k-1);
            omega0k = [zeros(3,3) , eye(3)]*Kinematics.Ji.Ji(:,:,k-1)*zeta;
            omegabk = omega0k - (Rbk')*omega0b;
            dJi(:,k) = [zeros(3,3), skew(dpbk)*Rbk*skew(omegabk) ...
                ; zeros(3,3) , (Rbk')*skew(omegabk)]*Xii;
       end
    end
    Ji=getji(Kinematics.Ti, i);
    Adg_inv = Kinematics.Ti.Adgbi_inv(:,:,i);
    Jgi_dot = [dAdg_inv, dAdg_inv*Ji + Adg_inv*dJi ];
end

function omegaib = getOmegaib(Kinematics,zeta,i)
% returns angular rage of vehcile wrt frame i noted in vehicle frame
    omegaib = zeros(3,1);
    Rbi = Kinematics.Ti.Rbi(:,:,i);
    Jgi = Kinematics.Ji.Ji(:,:,i);
    omega0b = zeta(4:6);
    omegaib = omega0b - Rbi*[zeros(3,3), eye(3)]*Jgi*zeta;
end

function dpbi = getDpbi( Kinematics, zeta,iter)
% returns time derivative of position vector of from frame b to frame i
    dpbi = zeros(3,1);
    H = [eye(3), zeros(3,3)];
    Rbi=Kinematics.Ti.Rbi(:,:,iter);
    Adgbi_inv = Kinematics.Ti.Adgbi_inv(:,:,iter);
    Ji = getji(Kinematics.Ti,iter);
    qd=zeros(6,1);
    qd(:,:)=zeta(7:12);
    dpbi = Rbi*H*Adgbi_inv*Ji*qd;
end


function mat = getji(Ti,i)
% return matrix Ji (see report)
    n=6;
    mat=zeros(6,6);
    Xii=[0,0,0,0,0,1]';
    mat(:,1)=eye(6)*Xii;
    for j=2:n
        if j<=i
            mat(:,j) = Ti.Adgbi(:,:,j-1)*Xii;
        end
    end
end


function S = skew(v)
  S = [  0   -v(3)  v(2)
       v(3)  0    -v(1)
       -v(2) v(1)   0];
end

== matlab function UVMS/Kinetics/Dynamics Matrices/getzeta ==
  data: Measured_States input double; zeta output double
function zeta = fcn(Measured_States)
%#codegen
    zeta = Measured_States.zeta;

end

== matlab function UVMS/Kinetics/Dynamics Matrices/Ma*H ==
  data: Measured_States input Bus: measured_states_bus; Kinetics_Parameters input double; MaH output double; zeta input double
function MaH = fcn(Measured_States,Kinetics_Parameters,zeta)
%#codegen ..........................
%
%  returns rest of the the added mass
%  force matrix:
%       Ma*H(xi,zeta)
% ..................................
    n=6;
    i=1;
    
    %% get the total Added mass matrix
    Ma = zeros(12,12);
    AddedInertia = Kinetics_Parameters.AddedInertia;
    Jgb = [eye(6), zeros(6,6)];                                 % Jacobian from vehicle 
    Ji=Jgb;
    Hi = Kinetics_Parameters.Persistent.Adgici(:,:,i);
    Ii=Hi'*( AddedInertia(:,:,1))*Hi;                           % Inertia of vehicle in CO
    Ma=Ma+(Ji')*Ii*Ji;
    for i=1:n
        Ji = Measured_States.Ji.Ji(:,:,i);                           % body jacobian
        Hi =Kinetics_Parameters.Persistent.Adgici(:,:,i+1);        % get Transformation matrix of link i
        Ii=Hi'*(AddedInertia(:,:,i+1))*Hi;                      % Transform Inertia matrix from CG to CO
        Ma=Ma+(Ji')*Ii*Ji;                                      % Add link i's inertia to total inertia
    end
    
    %% calculate the matrix product
    H = zeros(12,6);
    R0b = Measured_States.Ti.R0b;
    omega0b = zeta(4:6);
    H(1:3,1:3) = R0b'*skew(omega0b);
    MaH = Ma*H;
end

function S = skew(v)
  S = [  0   -v(3)  v(2)
       v(3)  0    -v(1)
       -v(2) v(1)   0];
end

== matlab function UVMS/Kinetics/Measure states/zeta2xi/zeta to dot xi ==
  data: zeta input double; dq output double; dp output double; dQ output double; Q input double
function [dq, dp, dQ] = fcn(zeta, Q)                       
    %#codegen
    R0b = Rquat(Q);
    U = getU(Q);
    Ja = [...
            R0b , zeros(3,3) , zeros(3,6);
            zeros(4, 3),  U,    zeros(4,6);
            zeros(6 ,6) , eye(6);
    ];
    
    dXi = Ja * zeta;
    dp = dXi(1:3);
    normalization_feedback = getNormalizationFeedback(Q);   % ensure that the quaternion is unit length
    dQ = dXi(4:7) + normalization_feedback;
    dq = dXi(8:13);
end





%----------------------------------------------------------------
%   use normalization feedback according to fossen
%   page 31 to ensure unity of quaternion
function qout = getNormalizationFeedback(qin)
    gamma = 100;
    qout = gamma*0.5*(1-qin'*qin)*qin;

end

%----------------------------------------------------------------
% get the transformation matrix for quaternions
function U = getU(Q)
    eta  = Q(1); eps1 = Q(2); eps2 = Q(3); eps3 = Q(4); 
    U = 0.5*[...
   -eps1 -eps2 -eps3        
    eta  -eps3  eps2
    eps3  eta  -eps1
   -eps2  eps1  eta   ];
end


function R = Rquat(q)
% R = Rquat(q) computes the quaternion rotation matrix R in SO(3)
% for q = [eta eps1 eps2 eps3]
%
% Author:    Thor I. Fossen
% Date:      14th June 2001
% Revisions: 6 October 2001, T I. Fossen - eta as first element in q  
% ________________________________________________________________
%
% MSS GNC is a Matlab toolbox for guidance, navigation and control.
% The toolbox is part of the Marine Systems Simulator (MSS).
%
% Copyright (C) 2008 Thor I. Fossen and Tristan Perez
% 
% This program is free software: you can redistribute it and/or modify
% it under the terms of the GNU General Public License as published by
% the Free Software Foundation, either version 3 of the License, or
% (at your option) any later version.
% 
% This program is distributed in the hope that it will be useful, but
% WITHOUT ANY WARRANTY; without even the implied warranty of
% MERCHANTABILITY or FITNESS FOR A PARTICULAR PURPOSE.  See the 
% GNU General Public License for more details.
% 
% You should have received a copy of the GNU General Public License
% along with this program.  If not, see <http://www.gnu.org/licenses/>.
% 
% E-mail: contact@marinecontrol.org
% URL:    <http://www.marinecontrol.org>

tol = 5*1e-2;
if abs(norm(q)-1)>tol
    q
    norm(q)
    error('Quaternion not unit. Norm(q) must be equal to 1 (in kinetics - measure states) Try decreasing the sampling rate'); 
end

eta = q(1);
eps = q(2:4);

S = Smtrx(eps);
R = eye(3) + 2*eta*S + 2*S^2;
end
